simulink model "TestHinf2States"  (R2020b)
settings: Solver=VariableStepAuto  StartTime=0.0  StopTime=10.0  RelTol=1e-3
undefined symbols (not defined in the file): act1, act2, Cd, k5, k6, k7, M, tfAct1, tfAct2
settings Model: Creator=jeremie  LastModifiedBy=jeremie
settings DebuggingCC: ArithmeticOperatorsInVariantConditions=warning
settings SFSimCC: CustomCodeUndefinedFunction=UseInterfaceOnly

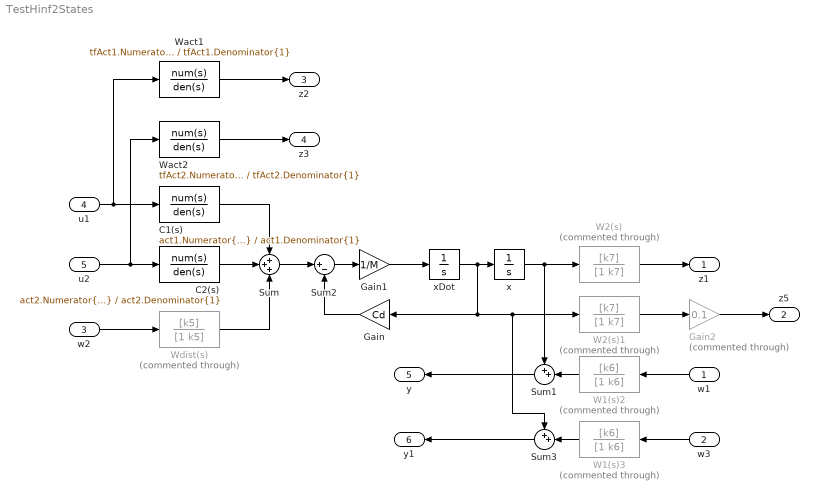
== system TestHinf2States ==
  w1 : Inport
  w3 : Inport  Port=2
  w2 : Inport  Port=3
  u1 : Inport  Port=4
  u2 : Inport  Port=5
  C1(s) : TransferFcn  Numerator=act1.Numerator{1}  Denominator=act1.Denominator{1}
  C2(s) : TransferFcn  Numerator=act2.Numerator{1}  Denominator=act2.Denominator{1}
  Gain : Gain  Gain=Cd
  Gain1 : Gain  Gain=1/M
  Gain2 : Gain  Commented=through  Gain=0.1
  Sum : Sum  Inputs=+++
  Sum1 : Sum  Inputs=++|
  Sum2 : Sum  Inputs=|+-
  Sum3 : Sum  Inputs=++|
  W1(s)2 : TransferFcn  Commented=through  Numerator=[k6]  Denominator=[1 k6]
  W1(s)3 : TransferFcn  Commented=through  Numerator=[k6]  Denominator=[1 k6]
  W2(s) : TransferFcn  Commented=through  Numerator=[k7]  Denominator=[1 k7]
  W2(s)1 : TransferFcn  Commented=through  Numerator=[k7]  Denominator=[1 k7]
  Wact1 : TransferFcn  Numerator=tfAct1.Numerator{1}  Denominator=tfAct1.Denominator{1}
  Wact2 : TransferFcn  Numerator=tfAct2.Numerator{1}  Denominator=tfAct2.Denominator{1}
  Wdist(s) : TransferFcn  Commented=through  Numerator=[k5]  Denominator=[1 k5]
  x : Integrator
  xDot : Integrator
  z1 : Outport  VectorParamsAs1DForOutWhenUnconnected=off
  z5 : Outport  Port=2  VectorParamsAs1DForOutWhenUnconnected=off
  z2 : Outport  Port=3  VectorParamsAs1DForOutWhenUnconnected=off
  z3 : Outport  Port=4  VectorParamsAs1DForOutWhenUnconnected=off
  y : Outport  Port=5  VectorParamsAs1DForOutWhenUnconnected=off
  y1 : Outport  Port=6  VectorParamsAs1DForOutWhenUnconnected=off
  wires:
  Sum/1 -> Sum2/1
  C2(s)/1 -> Sum/2
  C1(s)/1 -> Sum/1
  Wdist(s)/1 -> Sum/3
  x/1 -> W2(s)/1, Sum1/1
  W1(s)2/1 -> Sum1/2
  u2/1 -> Wact2/1, C2(s)/1
  u1/1 -> C1(s)/1, Wact1/1
  Wact1/1 -> z2/1
  W2(s)/1 -> z1/1
  w1/1 -> W1(s)2/1
  w2/1 -> Wdist(s)/1
  Sum1/1 -> y/1
  Wact2/1 -> z3/1
  Gain/1 -> Sum2/2
  Gain1/1 -> xDot/1
  Sum2/1 -> Gain1/1
  xDot/1 -> x/1, Gain/1, Sum3/1, W2(s)1/1
  W2(s)1/1 -> Gain2/1
  Sum3/1 -> y1/1
  w3/1 -> W1(s)3/1
  W1(s)3/1 -> Sum3/2
  Gain2/1 -> z5/1
